simulink model "RCRC"  (R2019a)
settings: Solver=VariableStepAuto  StartTime=0.0  StopTime=10.0  RelTol=1e-3
values from neighbouring files (symbols this model uses):
  C1 = 1    [value.m]
  C2 = 1    [value.m]
  R1 = 1    [value.m]
  R2 = 1    [value.m]
settings Model: Creator=Takumi SHIOTA  LastModifiedBy=Takumi SHIOTA

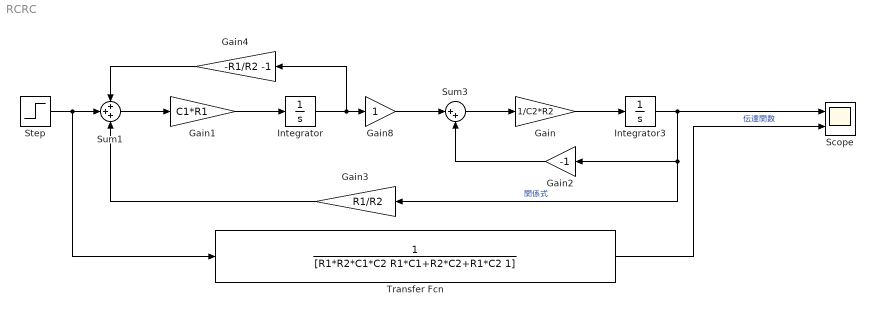
== system RCRC ==
  Gain : Gain  Gain=1/C2*R2
  Gain1 : Gain  Gain=C1*R1
  Gain2 : Gain  Gain=-1
  Gain3 : Gain  Gain=R1/R2
  Gain4 : Gain  Gain=-R1/R2 -1
  Gain8 : Gain
  Integrator : Integrator
  Integrator3 : Integrator
  Scope : Scope  NumInputPorts=2
  Step : Step  SampleTime=0
  Sum1 : Sum  Inputs=+++
  Sum3 : Sum  Inputs=|++
  Transfer Fcn : TransferFcn  Denominator=[R1*R2*C1*C2 R1*C1+R2*C2+R1*C2 1]
  wires:
  Sum3/1 -> Gain/1
  Sum1/1 -> Gain1/1
  Step/1 -> Sum1/2, Transfer Fcn/1
  Integrator3/1 -> Scope/1, Gain3/1, Gain2/1  "関係式"
  Gain/1 -> Integrator3/1
  Gain1/1 -> Integrator/1
  Integrator/1 -> Gain4/1, Gain8/1
  Gain2/1 -> Sum3/2
  Gain3/1 -> Sum1/3
  Gain4/1 -> Sum1/1
  Gain8/1 -> Sum3/1
  Transfer Fcn/1 -> Scope/2  "伝達関数"
